simulink model "bai311"  (R2022b)
settings: Solver=ode4  StartTime=0.0  StopTime=20  FixedStep=0.0001  RelTol=1e-8
undefined symbols (not defined in the file or in its folder): k
settings Model: Creator=ASUS  LastModifiedBy=admin

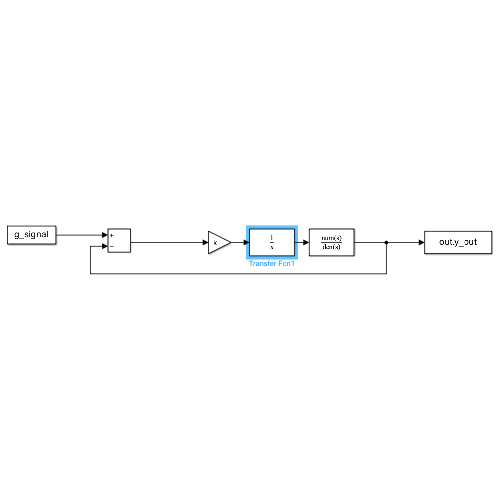
[thumbnail: Simulink's stored preview of the top-level diagram]
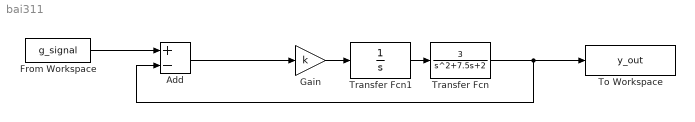
== system bai311 ==
  Add : Sum  Inputs=+-
  From Workspace : FromWorkspace  VariableName=g_signal
  Gain : Gain  Gain=k
  To Workspace : ToWorkspace  VariableName=y_out  SaveFormat=Structure With Time  SampleTime=-1
  Transfer Fcn : TransferFcn  Numerator=[3]  Denominator=[1 7.5 2]
  Transfer Fcn1 : TransferFcn  Denominator=[1 0]
  wires:
  From Workspace/1 -> Add/1
  Add/1 -> Gain/1
  Transfer Fcn/1 -> To Workspace/1, Add/2
  Gain/1 -> Transfer Fcn1/1
  Transfer Fcn1/1 -> Transfer Fcn/1
